simulink model "ACCLogic_Test"  (Simulink 7.8)
settings: Solver=ode3  StartTime=0.0  StopTime=35  FixedStep=TIMESTEP  RelTol=1e-3
InitFcn:
  | ACCLogic_TestCase2
StopFcn:
  | ACCLogic_plot
values from neighbouring files (symbols this model uses):
  H = 10    [parameters.m]
undefined symbols (not defined in the file or in its folder): Car1_start_s, Car1_us, Car2_start_s, Car2_us, Car3_start_s, Car3_us, Car4_start_s, Car4_us, Car5_start_s, Car5_us, ManEnt1, ManEnt2, ManEnt3, ManEnt4, MyCarMan_us, MyCarVel_us, TIMESTEP
libraries: simulink x5
settings Model: Creator=jmapatel  LastModifiedBy=Jesse Ku

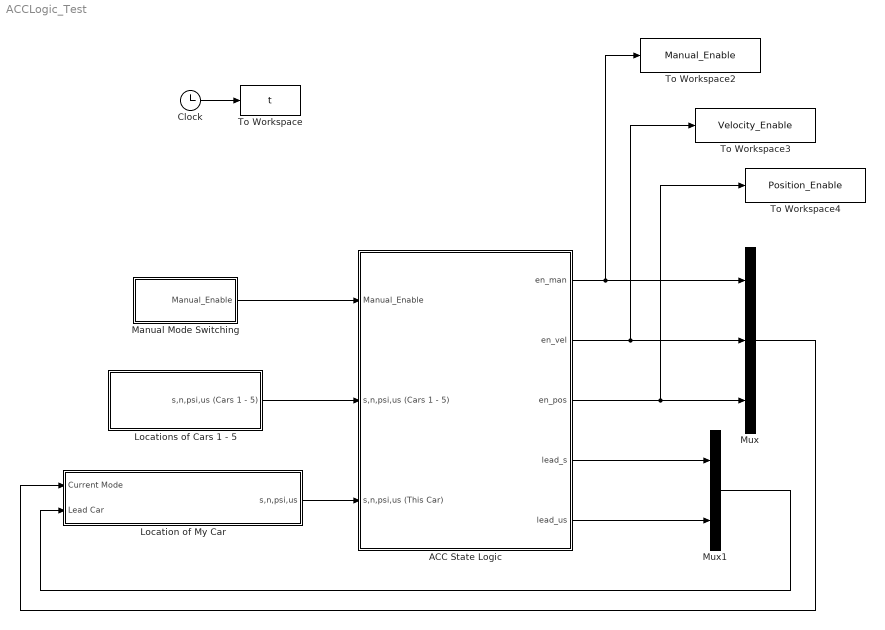
== system ACCLogic_Test ==
  ACC State Logic : Subsystem
  Clock : Clock
  Location of My Car : Subsystem
  Locations of Cars 1 - 5 : Subsystem
  Manual Mode Switching : Subsystem
  Mux : Mux  Inputs=3
  Mux1 : Mux  Inputs=2
  To Workspace : ToWorkspace  VariableName=t  SampleTime=-1  SaveFormat=Array
  To Workspace2 : ToWorkspace  VariableName=Manual_Enable  SampleTime=-1  SaveFormat=Array
  To Workspace3 : ToWorkspace  VariableName=Velocity_Enable  SampleTime=-1  SaveFormat=Array
  To Workspace4 : ToWorkspace  VariableName=Position_Enable  SampleTime=-1  SaveFormat=Array
  wires:
  Clock/1 -> To Workspace/1
  Manual Mode Switching/1(Manual_Enable) -> ACC State Logic/1(Manual_Enable)
  Locations of Cars 1 - 5/1(s,n,psi,us (Cars 1 - 5)) -> ACC State Logic/2(s,n,psi,us (Cars 1 - 5))
  Location of My Car/1(s,n,psi,us) -> ACC State Logic/3(s,n,psi,us (This Car))
  ACC State Logic/1(en_man) -> Mux/1, To Workspace2/1
  ACC State Logic/2(en_vel) -> Mux/2, To Workspace3/1
  ACC State Logic/3(en_pos) -> Mux/3, To Workspace4/1
  ACC State Logic/4(lead_s) -> Mux1/1
  ACC State Logic/5(lead_us) -> Mux1/2
  Mux/1 -> Location of My Car/1(Current Mode)
  Mux1/1 -> Location of My Car/2(Lead Car)

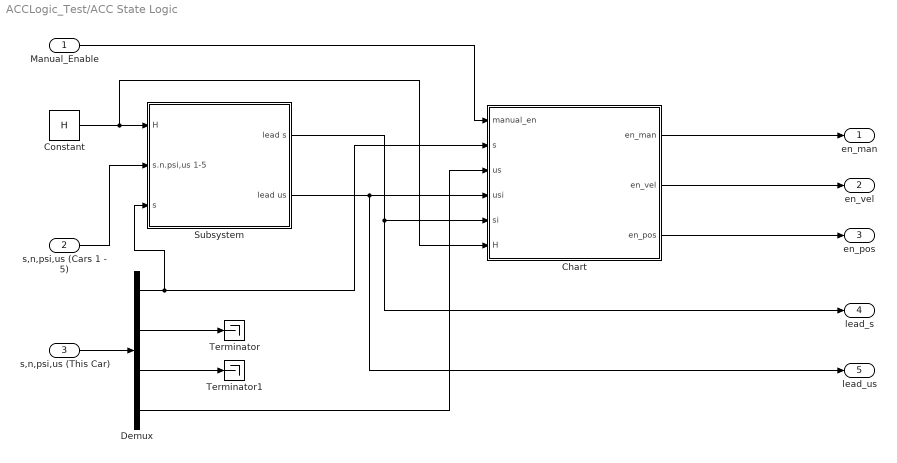
== system ACCLogic_Test/ACC State Logic ==
  Manual_Enable : Inport
  s,n,psi,us (Cars 1 - 5) : Inport  Port=2
  s,n,psi,us (This Car) : Inport  Port=3
  Chart : Stateflow chart  TreatAsAtomicUnit=on
  Constant : Constant  Value=H  OutDataTypeStr=single
  Demux : Demux
  Subsystem : Subsystem
  Terminator : Terminator
  Terminator1 : Terminator
  en_man : Outport
  en_vel : Outport  Port=2
  en_pos : Outport  Port=3
  lead_s : Outport  Port=4
  lead_us : Outport  Port=5
  wires:
  Constant/1 -> Subsystem/1(H), Chart/6(H)
  s,n,psi,us (Cars 1 - 5)/1 -> Subsystem/2(s.n.psi,us 1-5)
  s,n,psi,us (This Car)/1 -> Demux/1
  Demux/1 -> Chart/2(s), Subsystem/3(s)
  Demux/2 -> Terminator/1
  Demux/3 -> Terminator1/1
  Manual_Enable/1 -> Chart/1(manual_en)
  Subsystem/1(lead s) -> Chart/5(si), lead_s/1
  Subsystem/2(lead us) -> Chart/4(usi), lead_us/1
  Demux/4 -> Chart/3(us)
  Chart/1(en_man) -> en_man/1
  Chart/2(en_vel) -> en_vel/1
  Chart/3(en_pos) -> en_pos/1

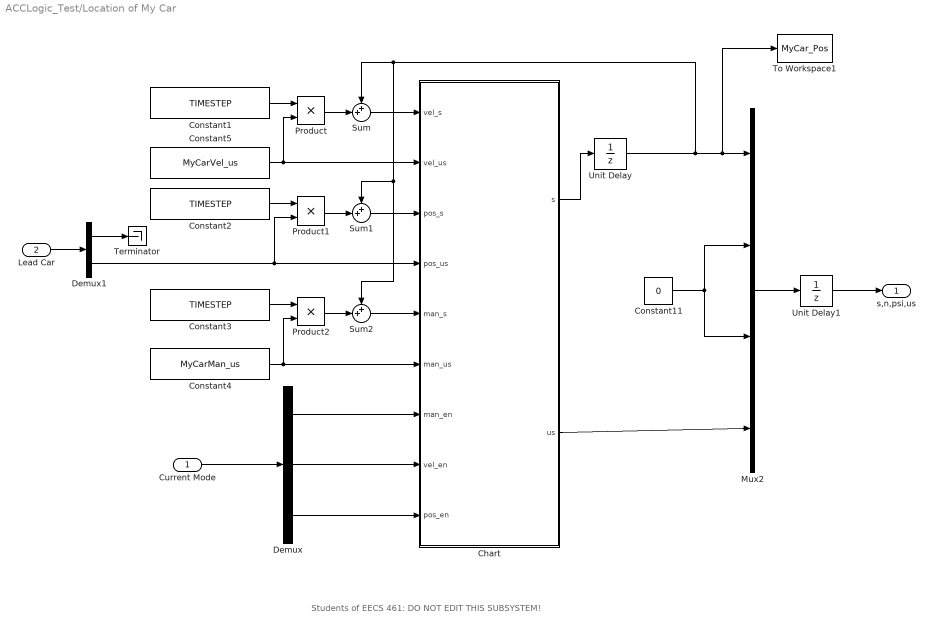
== system ACCLogic_Test/Location of My Car ==
  note: Students of EECS 461: DO NOT EDIT THIS SUBSYSTEM!
  Current Mode : Inport
  Lead Car : Inport  Port=2
  Chart : Stateflow chart  TreatAsAtomicUnit=on
  Constant1 : Constant  Value=TIMESTEP  OutDataTypeStr=single
  Constant11 : Constant  Value=0  OutDataTypeStr=single
  Constant2 : Constant  Value=TIMESTEP  OutDataTypeStr=single
  Constant3 : Constant  Value=TIMESTEP  OutDataTypeStr=single
  Constant4 : Constant  Value=MyCarMan_us  OutDataTypeStr=single
  Constant5 : Constant  Value=MyCarVel_us  OutDataTypeStr=single
  Demux : Demux  Outputs=3
  Demux1 : Demux  Outputs=2
  Mux2 : Mux
  Product : Product  RndMeth=Zero
  Product1 : Product  RndMeth=Zero
  Product2 : Product  RndMeth=Zero
  Sum : Sum  Inputs=++|
  Sum1 : Sum  Inputs=++|
  Sum2 : Sum  Inputs=++|
  Terminator : Terminator
  To Workspace1 : ToWorkspace  VariableName=MyCar_Pos  SampleTime=-1  SaveFormat=Array
  Unit Delay : UnitDelay  SampleTime=-1
  Unit Delay1 : UnitDelay  SampleTime=-1
  s,n,psi,us : Outport
  wires:
  Chart/2(us) -> Mux2/4
  Demux/1 -> Chart/7(man_en)
  Demux/2 -> Chart/8(vel_en)
  Demux/3 -> Chart/9(pos_en)
  Sum/1 -> Chart/1(vel_s)
  Product/1 -> Sum/2
  Constant1/1 -> Product/1
  Product1/1 -> Sum1/2
  Constant2/1 -> Product1/1
  Sum1/1 -> Chart/3(pos_s)
  Sum2/1 -> Chart/5(man_s)
  Product2/1 -> Sum2/2
  Constant3/1 -> Product2/1
  Chart/1(s) -> Unit Delay/1
  Unit Delay/1 -> Mux2/1, To Workspace1/1, Sum/1, Sum1/1, Sum2/1
  Mux2/1 -> Unit Delay1/1
  Unit Delay1/1 -> s,n,psi,us/1
  Current Mode/1 -> Demux/1
  Constant4/1 -> Chart/6(man_us), Product2/2
  Constant5/1 -> Chart/2(vel_us), Product/2
  Constant11/1 -> Mux2/2, Mux2/3
  Lead Car/1 -> Demux1/1
  Demux1/1 -> Terminator/1
  Demux1/2 -> Chart/4(pos_us), Product1/2

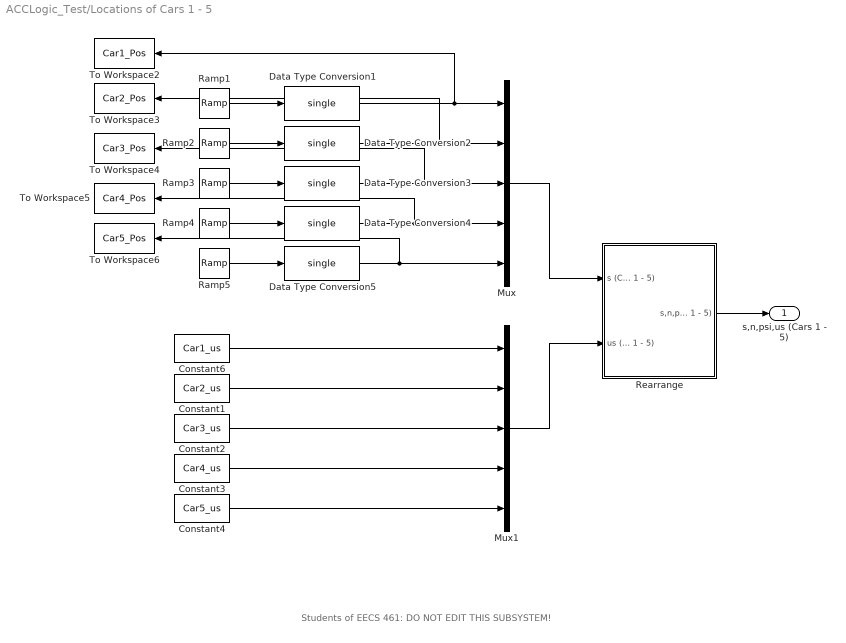
== system ACCLogic_Test/Locations of Cars 1 - 5 ==
  note: Students of EECS 461: DO NOT EDIT THIS SUBSYSTEM!
  Constant1 : Constant  Value=Car2_us  OutDataTypeStr=single
  Constant2 : Constant  Value=Car3_us  OutDataTypeStr=single
  Constant3 : Constant  Value=Car4_us  OutDataTypeStr=single
  Constant4 : Constant  Value=Car5_us  OutDataTypeStr=single
  Constant6 : Constant  Value=Car1_us  OutDataTypeStr=single
  Data Type Conversion{1..5} (5 alike) : DataTypeConversion  OutDataTypeStr=single
  Mux : Mux  Inputs=5
  Mux1 : Mux  Inputs=5
  Ramp1 : simulink/Sources/Ramp  slope=Car1_us  start=0  X0=Car1_start_s
  Ramp2 : simulink/Sources/Ramp  slope=Car2_us  start=0  X0=Car2_start_s
  Ramp3 : simulink/Sources/Ramp  slope=Car3_us  start=0  X0=Car3_start_s
  Ramp4 : simulink/Sources/Ramp  slope=Car4_us  start=0  X0=Car4_start_s
  Ramp5 : simulink/Sources/Ramp  slope=Car5_us  start=0  X0=Car5_start_s
  Rearrange : Subsystem
  To Workspace2 : ToWorkspace  VariableName=Car1_Pos  SampleTime=-1  SaveFormat=Array
  To Workspace3 : ToWorkspace  VariableName=Car2_Pos  SampleTime=-1  SaveFormat=Array
  To Workspace4 : ToWorkspace  VariableName=Car3_Pos  SampleTime=-1  SaveFormat=Array
  To Workspace5 : ToWorkspace  VariableName=Car4_Pos  SampleTime=-1  SaveFormat=Array
  To Workspace6 : ToWorkspace  VariableName=Car5_Pos  SampleTime=-1  SaveFormat=Array
  s,n,psi,us (Cars 1 - 5) : Outport
  wires:
  Constant6/1 -> Mux1/1
  Constant1/1 -> Mux1/2
  Constant2/1 -> Mux1/3
  Constant3/1 -> Mux1/4
  Constant4/1 -> Mux1/5
  Mux/1 -> Rearrange/1(s (Cars 1 - 5))
  Mux1/1 -> Rearrange/2(us (Cars 1 - 5))
  Ramp1/1 -> Data Type Conversion1/1
  Data Type Conversion1/1 -> Mux/1, To Workspace2/1
  Ramp2/1 -> Data Type Conversion2/1
  Data Type Conversion2/1 -> Mux/2, To Workspace3/1
  Ramp3/1 -> Data Type Conversion3/1
  Data Type Conversion3/1 -> Mux/3, To Workspace4/1
  Ramp4/1 -> Data Type Conversion4/1
  Data Type Conversion4/1 -> Mux/4, To Workspace5/1
  Ramp5/1 -> Data Type Conversion5/1
  Data Type Conversion5/1 -> Mux/5, To Workspace6/1
  Rearrange/1(s,n,psi,us (Cars 1 - 5)) -> s,n,psi,us (Cars 1 - 5)/1

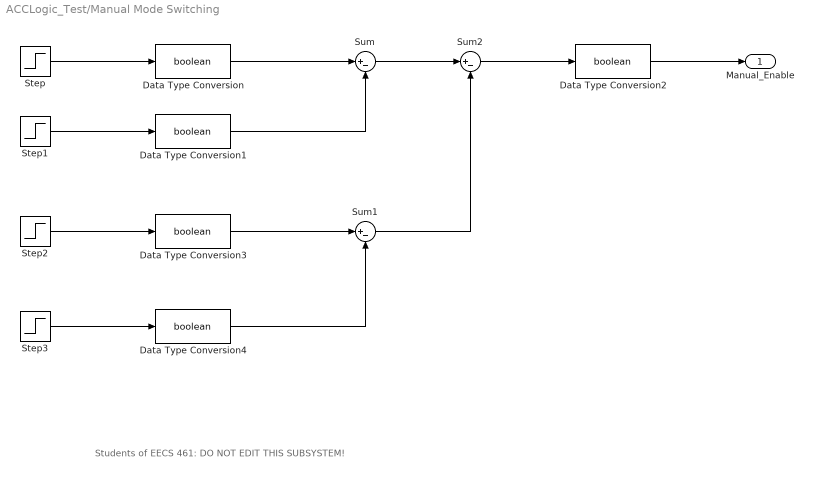
== system ACCLogic_Test/Manual Mode Switching ==
  note: Students of EECS 461: DO NOT EDIT THIS SUBSYSTEM!
  Data Type Conversion{,1..4} (5 alike) : DataTypeConversion  OutDataTypeStr=boolean
  Step : Step  Time=ManEnt1  SampleTime=0
  Step1 : Step  Time=ManEnt2  SampleTime=0
  Step2 : Step  Time=ManEnt3  SampleTime=0
  Step3 : Step  Time=ManEnt4  SampleTime=0
  Sum : Sum  Inputs=|+-
  Sum1 : Sum  Inputs=|+-
  Sum2 : Sum  Inputs=|+-
  Manual_Enable : Outport
  wires:
  Step/1 -> Data Type Conversion/1
  Step1/1 -> Data Type Conversion1/1
  Data Type Conversion/1 -> Sum/1
  Data Type Conversion1/1 -> Sum/2
  Data Type Conversion2/1 -> Manual_Enable/1
  Step2/1 -> Data Type Conversion3/1
  Step3/1 -> Data Type Conversion4/1
  Data Type Conversion3/1 -> Sum1/1
  Data Type Conversion4/1 -> Sum1/2
  Sum/1 -> Sum2/1
  Sum1/1 -> Sum2/2
  Sum2/1 -> Data Type Conversion2/1

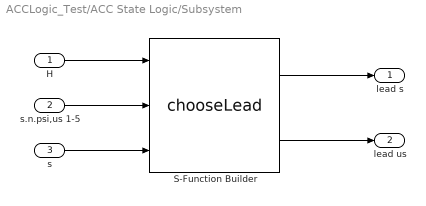
== system ACCLogic_Test/ACC State Logic/Subsystem ==
  H : Inport
  s.n.psi,us 1-5 : Inport  Port=2
  s : Inport  Port=3
  S-Function Builder : S-Function  InitFcn=try, set_param(gcb,'FunctionName','chooseLead'), end  FunctionName=chooseLead  SFunctionModules=chooseLead_wrapper  WizardData=DataTag0  EnableBusSupport=off  mask(S-Function Builder){}
      mask help: Simulink:masks:SFunctionBuilder_MD
      mask init:
      | val = [[.9  0.75 0.75 1 1 .9 .9 1]',[1 1 0.75 0.75 .9 .9 1 .9]'];try , sys = get_param(gcb,'SfunBuilderFcnName');if isempty(sys), sys = get_param(gcb,'FunctionName'); end,catch, sys = get_param(gcb,'FunctionName'); end
      settings: CopyFcn=set_param(gcbh,'LinkStatus','none')  PreSaveFcn=try, set_param(gcb,'FunctionName','chooseLead'), end  OpenFcn=sfunctionwizard(gcbh)
      mask Display:
      | plot(val(:,1),val(:,2))
      | disp(sys)
      | port_label('input',1,'H')
      | port_label('input',2,'in')
      | port_label('input',3,'s')
      | port_label('output',1,'si')
      | port_label('output',2,'usi')
  lead s : Outport
  lead us : Outport  Port=2
  wires:
  s.n.psi,us 1-5/1 -> S-Function Builder/2
  H/1 -> S-Function Builder/1
  s/1 -> S-Function Builder/3
  S-Function Builder/1 -> lead s/1
  S-Function Builder/2 -> lead us/1

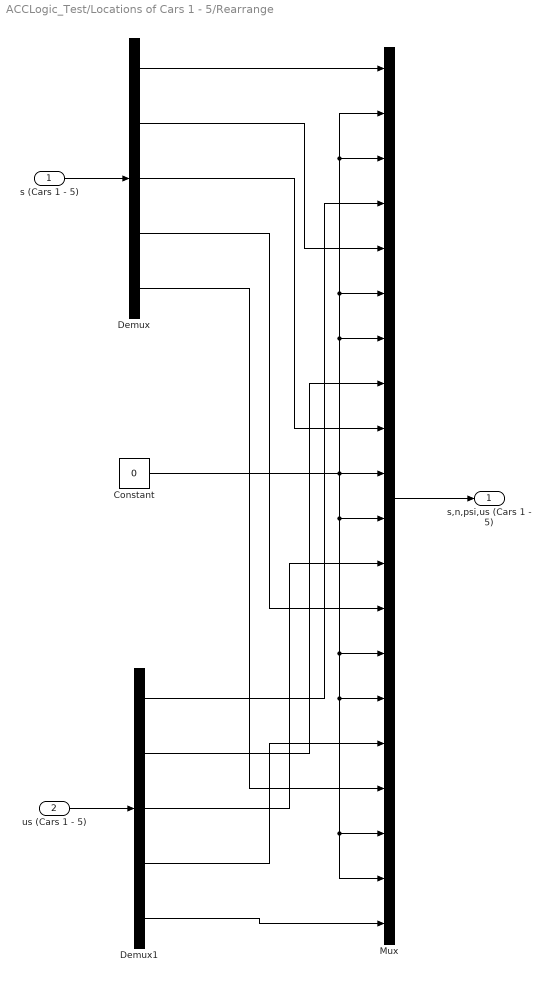
== system ACCLogic_Test/Locations of Cars 1 - 5/Rearrange ==
  s (Cars 1 - 5) : Inport
  us (Cars 1 - 5) : Inport  Port=2
  Constant : Constant  Value=0  OutDataTypeStr=single
  Demux : Demux  Outputs=5
  Demux1 : Demux  Outputs=5
  Mux : Mux  Inputs=20
  s,n,psi,us (Cars 1 - 5) : Outport
  wires:
  us (Cars 1 - 5)/1 -> Demux1/1
  s (Cars 1 - 5)/1 -> Demux/1
  Demux/1 -> Mux/1
  Constant/1 -> Mux/2, Mux/3, Mux/6, Mux/7, Mux/10, Mux/11, Mux/19, Mux/18, Mux/15, Mux/14
  Demux1/1 -> Mux/4
  Demux/2 -> Mux/5
  Demux1/2 -> Mux/8
  Demux/3 -> Mux/9
  Demux1/3 -> Mux/12
  Demux/4 -> Mux/13
  Demux1/4 -> Mux/16
  Demux/5 -> Mux/17
  Demux1/5 -> Mux/20
  Mux/1 -> s,n,psi,us (Cars 1 - 5)/1

== stateflow chart ACC State Logic/Chart ==
  state Position
    during:
    en_man = 0;
    en_vel = 0;
    en_pos = 1;
  state Velocity
    during:
    en_man = 0;
    en_vel = 1;
    en_pos = 0;
  state Manual
    during:
    en_man = 1;
    en_vel = 0;
    en_pos = 0;
  Position -> Manual [order 1] : [manual_en == 1]
  Velocity -> Manual [order 1] : [manual_en == 1]
  (default) -> Manual
  Velocity -> Position [order 2] : [((usi <= us) && ((si-s)<=H))]
  Position -> Velocity [order 2] : [((usi > us) || ((si-s) > H))]
  Manual -> Velocity : [manual_en != 1]
  data: manual_en input boolean; s input single; us input single; usi input single; si input single; H input single; en_man output boolean; en_vel output boolean; en_pos output boolean

== stateflow chart Location of My Car/Chart ==
  state vel_ctrl
    during:s = vel_s
    during:us = vel_us
  state pos_ctrl
    during:s = pos_s
    during:us = pos_us
  state man_ctrl
    during:s = man_s
    during:us = man_us
  vel_ctrl -> pos_ctrl [order 1] : [(pos_en==1)&(vel_en==0)&(man_en==0)]
  pos_ctrl -> vel_ctrl [order 1] : [(pos_en == 0)&(vel_en == 1)&(man_en == 0)]
  pos_ctrl -> man_ctrl [order 2] : [(pos_en == 0)&(vel_en == 0)&(man_en == 1)]
  man_ctrl -> pos_ctrl [order 1] : [(pos_en == 1)&(vel_en == 0)&(man_en == 0)]
  man_ctrl -> vel_ctrl [order 2] : [(pos_en == 0)&(vel_en == 1)&(man_en == 0)]
  vel_ctrl -> man_ctrl [order 2] : [(pos_en == 0)&(vel_en == 0)&(man_en == 1)]
  (default) -> vel_ctrl
  data: vel_s input single; vel_us input single; pos_s input single; pos_us input single; man_s input single; man_us input single; man_en input boolean; vel_en input boolean; pos_en input boolean; s output single; us output single
